simulink model "line_follower_robot"  (R2024b)
settings: Solver=ode4  StartTime=0.0  StopTime=P.T_sim  FixedStep=P.dt  RelTol=1e-3
undefined symbols (not defined in the file or in its folder): P
libraries: slpidlib x1
settings Model: Creator=vincent  LastModifiedBy=vincent

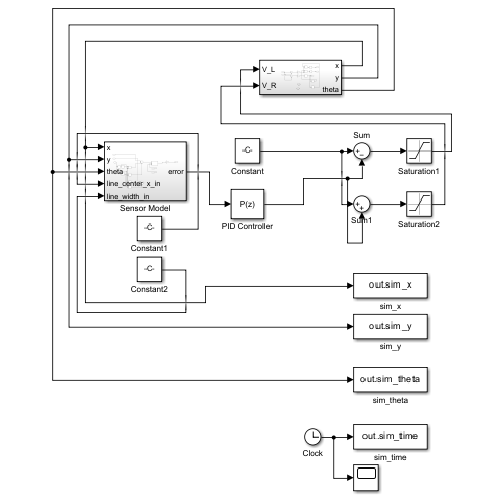
[thumbnail: Simulink's stored preview of the top-level diagram]
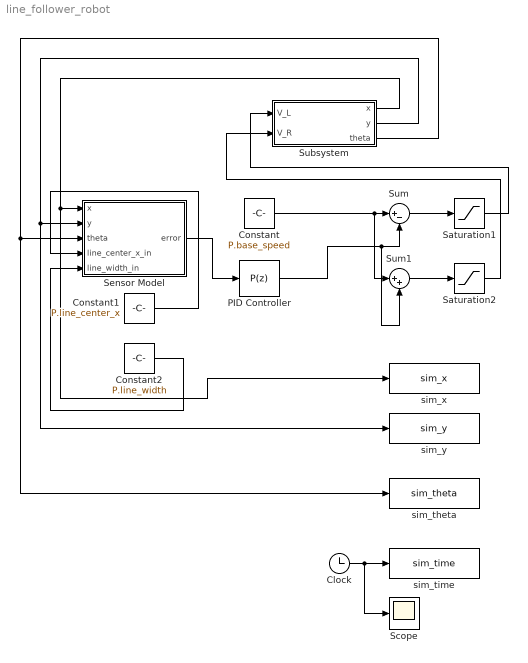
== system line_follower_robot ==
  Clock : Clock
  Constant : Constant  Value=P.base_speed
  Constant1 : Constant  Value=P.line_center_x
  Constant2 : Constant  Value=P.line_width
  PID Controller : slpidlib/PID Controller  Controller=P  Form=Parallel  TimeDomain=Discrete-time  UseExternalTs=off  SampleTime=P.dt  IntegratorMethod=Forward Euler  FilterMethod=Forward Euler  ControllerParametersSource=internal  P=P.Kp  I=1  UseKiTs=off  D=0  UseExternalDerivativeSource=off  N=100  UseFilter=on  TunerSelectOption=Transfer Function Based (PID Tuner App)  InitialConditionSource=internal  InitialConditionForIntegrator=0  InitialConditionForFilter=0  DifferentiatorICPrevScaledInput=0  ExternalReset=none  TrackingMode=off  Kt=1  LimitOutput=off  SatLimitsSource=internal  UpperSaturationLimit=inf  LowerSaturationLimit=-inf  LinearizeAsGain=on  AntiWindupMode=none  Kb=1  LimitIntegrator=off  UpperIntegratorSaturationLimit=inf  LowerIntegratorSaturationLimit=-inf  POutMin=[]  POutMax=[]  IOutMin=[]  IOutMax=[]  DOutMin=[]  DOutMax=[]  NOutMin=[]  NOutMax=[]  SumOutMin=[]  SumOutMax=[]  SaturationOutMin=[]  SaturationOutMax=[]  PParamMin=[]  PParamMax=[]  IParamMin=[]  IParamMax=[]  DParamMin=[]  DParamMax=[]  NParamMin=[]  NParamMax=[]  KbParamMin=[]  KbParamMax=[]  KtParamMin=[]  KtParamMax=[]  KbOutMin=[]  KbOutMax=[]  KtOutMin=[]  KtOutMax=[]  IntegratorOutMin=[]  IntegratorOutMax=[]  FilterOutMin=[]  FilterOutMax=[]  SumI1OutMin=[]  SumI1OutMax=[]  SumI2OutMin=[]  SumI2OutMax=[]  SumI3OutMin=[]  SumI3OutMax=[]  SumI4OutMin=[]  SumI4OutMax=[]  SumDOutMin=[]  SumDOutMax=[]  DifferentiatorOutMin=[]  DifferentiatorOutMax=[]  FilterDiffOutCoefMin=[]  FilterDiffOutCoefMax=[]  ReciprocalOutMin=[]  ReciprocalOutMax=[]  SumDenOutMin=[]  SumDenOutMax=[]  SumNumOutMin=[]  SumNumOutMax=[]  DivideOutMin=[]  DivideOutMax=[]  UdiffTsProdOutMin=[]  UdiffTsProdOutMax=[]  NTsProdOutMin=[]  NTsProdOutMax=[]  UintegralTsProdOutMin=[]  UintegralTsProdOutMax=[]  UngainTsProdOutMin=[]  UngainTsProdOutMax=[]  ClampingZeroOutDataTypeStr=Inherit: Inherit via back propagation  ClampingZeroOutMin=[]  ClampingZeroOutMax=[]  FilterDenConstantOutDataTypeStr=Inherit: Inherit via back propagation  FilterDenConstantOutMin=[]  FilterDenConstantOutMax=[]  PCopyOutDataTypeStr=Inherit: Inherit via back propagation  PCopyOutMin=[]  PCopyOutMax=[]  NCopyOutDataTypeStr=Inherit: Inherit via back propagation  NCopyOutMin=[]  NCopyOutMax=[]  IntegratorContinuousStateAttributes=''  IntegratorStateMustResolveToSignalObject=off  IntegratorRTWStateStorageClass=Auto  FilterContinuousStateAttributes=''  FilterStateMustResolveToSignalObject=off  FilterRTWStateStorageClass=Auto  ParallelPVariant=InternalParameters  IdealPVariant=Disabled  IVariant=Disabled  DVariant=Disabled  IntegratorVariant=Disabled  SatVariant=Disabled  AWVariant=Disabled  PCopyVariant=Disabled  TRVariant=Disabled  FdbkBlocksVariant=Forward  IdealPFdbkVariant=Disabled  SatFdbkVariant=Disabled  DerivativeFilterVariant=Disabled  NVariant=Disabled  NCopyVariant=Disabled_SignalSpec  FilterICVariant=Disabled  IntegratorICVariant=Disabled  ExternalResetVariant=Disabled  TRSumVariant=Passthrough  SumFdbkVariant=Disabled  SumVariant=Passthrough_P  TsampFilterVariant=InternalTs  TsampNgainVariant=Passthrough  TsampIntegralVariant=Disabled_SignalSpec  ExternalSaturationOutDataTypeStr=Inherit: Same as second input  DerivativeSourceVariant=Disabled  PreIntVariant=InternalPreInt
  Saturation1 : Saturate  UpperLimit=P.base_speed * 2  LowerLimit=P.base_speed
  Saturation2 : Saturate  UpperLimit=P.base_speed * 2  LowerLimit=P.base_speed
  Scope : Scope
  Sensor Model : Subsystem
  Subsystem : Subsystem
  Sum : Sum  Inputs=|+-
  Sum1 : Sum  Inputs=|++
  sim_theta : ToWorkspace  VariableName=sim_theta  SampleTime=-1
  sim_time : ToWorkspace  VariableName=sim_time  SampleTime=-1
  sim_x : ToWorkspace  VariableName=sim_x  SampleTime=-1
  sim_y : ToWorkspace  VariableName=sim_y  SampleTime=-1
  wires:
  Constant/1 -> Sum1/1, Sum/1
  PID Controller/1 -> Sum/2, Sum1/2
  Sum/1 -> Saturation1/1
  Sum1/1 -> Saturation2/1
  Saturation1/1 -> Subsystem/1(V_L)
  Saturation2/1 -> Subsystem/2(V_R)
  Sensor Model/1(error) -> PID Controller/1
  Subsystem/1(x) -> sim_x/1, Sensor Model/1(x)
  Subsystem/2(y) -> sim_y/1, Sensor Model/2(y)
  Subsystem/3(theta) -> sim_theta/1, Sensor Model/3(theta)
  Clock/1 -> sim_time/1, Scope/1
  Constant1/1 -> Sensor Model/4(line_center_x_in)
  Constant2/1 -> Sensor Model/5(line_width_in)

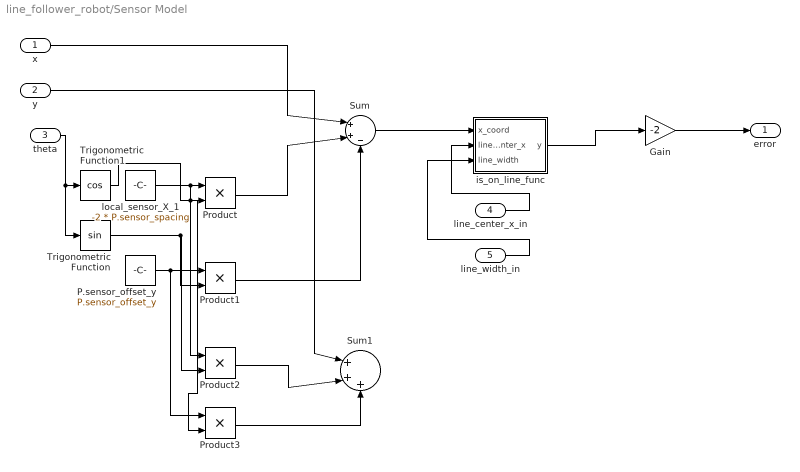
== system line_follower_robot/Sensor Model ==
  x : Inport
  y : Inport  Port=2
  theta : Inport  Port=3
  line_center_x_in : Inport  Port=4
  line_width_in : Inport  Port=5
  Gain : Gain  Gain=-2
  P.sensor_offset_y : Constant  Value=P.sensor_offset_y
  Product{,1..3} (4 alike) : Product
  Sum : Sum  Inputs=|++-
  Sum1 : Sum  Inputs=|+++
  Trigonometric Function : Trigonometry
  Trigonometric Function1 : Trigonometry  Operator=cos
  is_on_line_func : MATLAB Function  TreatAsAtomicUnit=on
  local_sensor_X_1 : Constant  Value=-2 * P.sensor_spacing
  error : Outport
  wires:
  theta/1 -> Trigonometric Function/1, Trigonometric Function1/1
  local_sensor_X_1/1 -> Product2/1, Product/1
  Trigonometric Function1/1 -> Product3/2, Product/2
  P.sensor_offset_y/1 -> Product1/1, Product3/1
  Trigonometric Function/1 -> Product2/2, Product1/2
  x/1 -> Sum/1
  Product/1 -> Sum/2
  Product1/1 -> Sum/3
  y/1 -> Sum1/1
  Product2/1 -> Sum1/2
  Product3/1 -> Sum1/3
  Sum/1 -> is_on_line_func/1(x_coord)
  is_on_line_func/1(y) -> Gain/1
  Gain/1 -> error/1
  line_center_x_in/1 -> is_on_line_func/2(line_center_x)
  line_width_in/1 -> is_on_line_func/3(line_width)

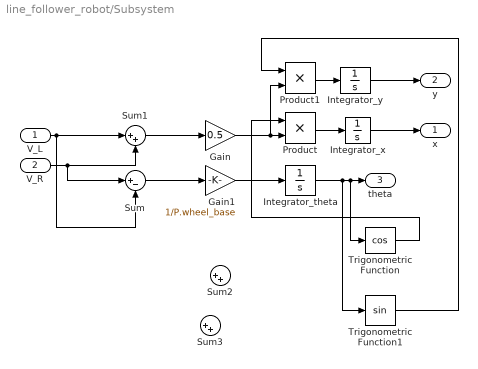
== system line_follower_robot/Subsystem ==
  V_L : Inport
  V_R : Inport  Port=2
  Gain : Gain  Gain=0.5
  Gain1 : Gain  Gain=1/P.wheel_base
  Integrator_theta : Integrator  InitialCondition=P.robot_theta0
  Integrator_x : Integrator  InitialCondition=P.robot_x0
  Integrator_y : Integrator  InitialCondition=P.robot_y0
  Product : Product
  Product1 : Product
  Sum : Sum  Inputs=|+-
  Sum1 : Sum  Inputs=|++
  Sum2 : Sum  Inputs=|++
  Sum3 : Sum  Inputs=|++
  Trigonometric Function : Trigonometry  Operator=cos
  Trigonometric Function1 : Trigonometry
  x : Outport
  y : Outport  Port=2
  theta : Outport  Port=3
  wires:
  V_L/1 -> Sum/2, Sum1/1
  V_R/1 -> Sum/1, Sum1/2
  Sum1/1 -> Gain/1
  Sum/1 -> Gain1/1
  Gain1/1 -> Integrator_theta/1
  Integrator_theta/1 -> Trigonometric Function/1, theta/1, Trigonometric Function1/1
  Gain/1 -> Product1/2, Product/2
  Trigonometric Function/1 -> Product/1
  Product/1 -> Integrator_x/1
  Integrator_x/1 -> x/1
  Trigonometric Function1/1 -> Product1/1
  Product1/1 -> Integrator_y/1
  Integrator_y/1 -> y/1

== matlab function line_follower_robot/Sensor Model/is_on_line_func ==
  data: x_coord input; y output; line_center_x input; line_width input
function y = is_on_line_func(x_coord, line_center_x, line_width)
% This block calculates if a point is on the line for code generation.

% Initialize the output variable 'y' to ensure it's always defined
% This line is CRUCIAL and must be the first executable line after the function definition.
y = 0;

if abs(x_coord - line_center_x) < line_width / 2
    y = 1; % Assign y a value if the condition is true
end

% No 'else' block is needed if 'y' is initialized to 0 and only changed to 1.
% If the 'if' condition is false, 'y' remains its initialized value of 0.
